simulink model "Quadcopter_NMPC_1"  (R2023a)
settings: Solver=VariableStepAuto  StartTime=0.0  StopTime=10.0  RelTol=1e-3
values from neighbouring files (symbols this model uses):
  Ts = 0.1    [ControlOfQuadrotorUsingNLMPCExample222.m]
undefined symbols (not defined in the file or in its folder): sigbuilder_block, v0, v_set
libraries: mpclib x3, sharedTrackingLibrary x2
settings Model: Creator=Hameed  LastModifiedBy=Hameed
settings DebuggingCC: UnconnectedInputMsg=warning  UnconnectedOutputMsg=warning  UnconnectedLineMsg=warning
settings ModelReferenceCC: EnableRefExpFcnMdlSchedulingChecks=on
settings RTWCC: DLArmComputeVersion=19.05

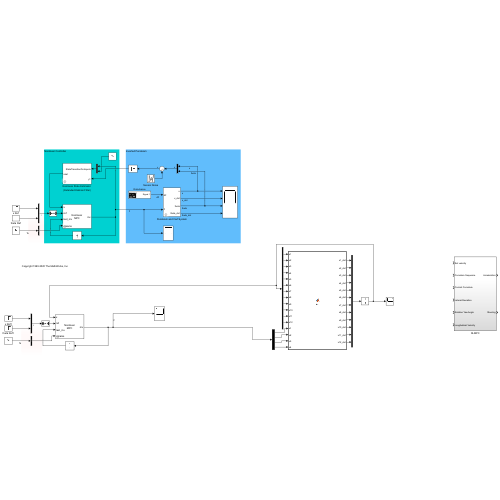
[thumbnail: Simulink's stored preview of the top-level diagram]
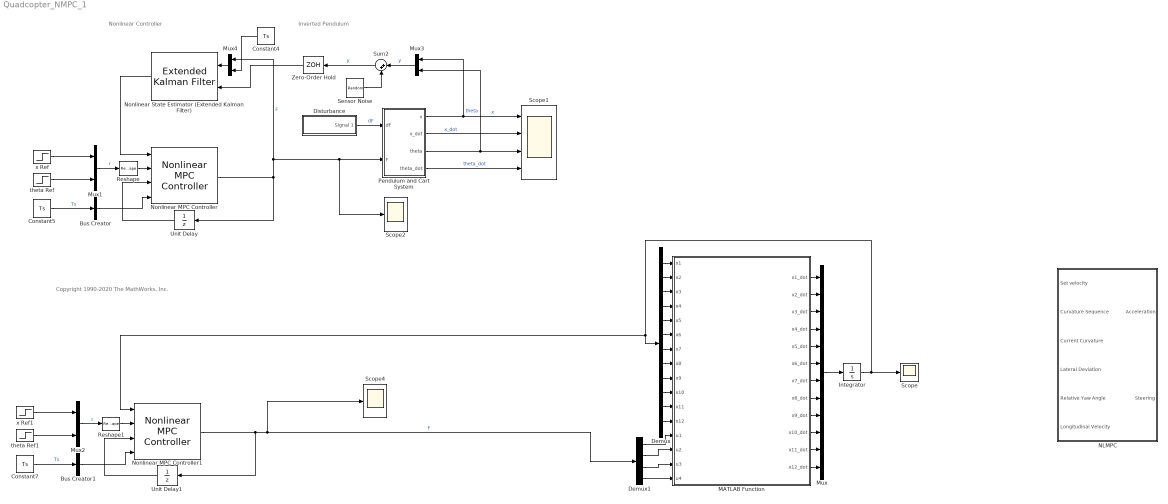
== system Quadcopter_NMPC_1 ==
  note: Inverted Pendulum
  note: Copyright 1990-2020 The MathWorks, Inc.
  note: Nonlinear Controller
  Bus Creator : BusCreator  Inputs=1  OutDataTypeStr=Bus: myBusObject  NonVirtualBus=on
      settings: InheritFromInputs=off
  Bus Creator1 : BusCreator  Inputs=1  OutDataTypeStr=Bus: myBusObject  NonVirtualBus=on
      settings: InheritFromInputs=off
  Constant4 : Constant  Value=Ts
  Constant5 : Constant  Value=Ts
  Constant7 : Constant  Value=Ts
  Demux : Demux  Outputs=12
  Demux1 : Demux
  Disturbance : Subsystem  Tag=STV Subsys  LoadFcn=sigbuilder_block('load');  StartFcn=sigbuilder_block('start');  StopFcn=sigbuilder_block('stop');  ClipboardFcn=sigbuilder_block('clipboard');  mask(Sigbuilder block){tuvar=[0:10]}
      mask help: Simulink:masks:SigbuilderBlock_MD
      mask init:
      | if ~strcmp(get_param(bdroot(gcbh),'SimulationStatus'),'stopped') tuvar = sigbuilder_block('maskInit'); end
      settings: CopyFcn=sigbuilder_block('copy');  DeleteFcn=sigbuilder_block('delete');  ModelCloseFcn=sigbuilder_block('modelClose');  PreSaveFcn=sigbuilder_block('preSave');  PauseFcn=sigbuilder_block('pause');  ContinueFcn=sigbuilder_block('continue');  NameChangeFcn=sigbuilder_block('namechange');  OpenFcn=sigbuilder_block('open',[237 156.75 551.25 355.5 ]);  CloseFcn=sigbuilder_block('close');
      mask Display: plot(0, 0, 100, 100,[2, 2, 32, 32, 2], [68, 8, 8, 68, 68],[32, 2], [38, 38], [32, 19, 2],[53, 60, 44], [32, 17, 17, 2],[16, 16, 31, 31]);txt = getActiveGroup(gcbh);text(2, 100, txt,'verticalAlignment', 'top');
  Integrator : Integrator  InitialCondition=[0;0;0;0;0;0;0;0;0;0;0;0]
  MATLAB Function : MATLAB Function  TreatAsAtomicUnit=on
  Mux : Mux  Inputs=12
  Mux{1..4} (4 alike) : Mux  Inputs=2
  NLMPC : Subsystem  VariantControl=controller_type ==1
  Nonlinear MPC Controller : mpclib/Nonlinear MPC Controller  SCDEnableBlockLinearizationSpecification=on  nlmpcobj=nlobj  UseObjectTs=on  UseMEX=off  md_enabled=off  mvtarget_enabled=off  param_enabled=on  cost_enabled=off  mvseq_enabled=off  stateseq_enabled=off  ovseq_enabled=off  slack_enabled=off  status_enabled=off  ov_min=off  ov_max=off  mv_min=off  mv_max=off  mvrate_min=off  mvrate_max=off  state_min=off  state_max=off  ov_weight=off  mv_weight=off  mvrate_weight=off  ecr_weight=off  nlp_initialize=off
  Nonlinear MPC Controller1 : mpclib/Nonlinear MPC Controller  SCDEnableBlockLinearizationSpecification=on  nlmpcobj=nlobj  UseObjectTs=on  UseMEX=off  md_enabled=off  mvtarget_enabled=off  param_enabled=on  cost_enabled=off  mvseq_enabled=off  stateseq_enabled=off  ovseq_enabled=off  slack_enabled=off  status_enabled=off  ov_min=off  ov_max=off  mv_min=off  mv_max=off  mvrate_min=off  mvrate_max=off  state_min=off  state_max=off  ov_weight=off  mv_weight=off  mvrate_weight=off  ecr_weight=off  nlp_initialize=off
  Nonlinear State Estimator (Extended Kalman Filter) : sharedTrackingLibrary/Extended Kalman Filter  StateTransitionFcn=pendulumStateFcn  HasStateTransitionJacobianFcn=off  HasAdditiveProcessNoise=Additive  ProcessNoise=1e-4*eye(4)  HasTimeVaryingProcessNoise=off  HasStateTransitionFcnExtraArgument=1  InitialState=[0;0;-pi;0]  InitialStateCovariance=1e-4*eye(4)  MeasurementFcn1=pendulumMeasurementFcn  HasMeasurementJacobianFcn1=off  HasMeasurementEnablePort1=off  HasAdditiveMeasurementNoise1=Additive  MeasurementNoise1=1e-4*eye(2)  HasTimeVaryingMeasurementNoise1=off  HasMeasurementFcnExtraArgument1=0  HasMeasurementWrapping1=off  MeasurementFcn2=myMeasurementFcn  HasMeasurementJacobianFcn2=off  HasMeasurementEnablePort2=off  HasAdditiveMeasurementNoise2=Additive  MeasurementNoise2=1  HasTimeVaryingMeasurementNoise2=off  HasMeasurementFcnExtraArgument2=0  HasMeasurementWrapping2=off  MeasurementFcn3=myMeasurementFcn  HasMeasurementJacobianFcn3=off  HasMeasurementEnablePort3=off  HasAdditiveMeasurementNoise3=Additive  MeasurementNoise3=1  HasTimeVaryingMeasurementNoise3=off  HasMeasurementFcnExtraArgument3=0  HasMeasurementWrapping3=off  MeasurementFcn4=myMeasurementFcn  HasMeasurementJacobianFcn4=off  HasMeasurementEnablePort4=off  HasAdditiveMeasurementNoise4=Additive  MeasurementNoise4=1  HasTimeVaryingMeasurementNoise4=off  HasMeasurementFcnExtraArgument4=0  HasMeasurementWrapping4=off  MeasurementFcn5=myMeasurementFcn  HasMeasurementJacobianFcn5=off  HasMeasurementEnablePort5=off  HasAdditiveMeasurementNoise5=Additive  MeasurementNoise5=1  HasTimeVaryingMeasurementNoise5=off  HasMeasurementFcnExtraArgument5=0  HasMeasurementWrapping5=off  EnableMultirate=off  StateTransitionFcnSampleTime=1  MeasurementFcn1SampleTime=1  MeasurementFcn2SampleTime=1  MeasurementFcn3SampleTime=1  MeasurementFcn4SampleTime=1  MeasurementFcn5SampleTime=1  UseCurrentEstimator=on  OutputStateCovariance=off  DataType=double  SampleTime=Ts  NumberOfMeasurements=1
  Pendulum and Cart System : Subsystem  mask{mCartPara=1, mPendPara=1, gPara=9.81, LPara=0.5, KdPara=10, x0=0, theta0=-pi}
      mask prompts: mCartPara "Mass of Cart"; mPendPara "Mass of Pendulum"; gPara "Gravity"; LPara "Length of Pendulum"; KdPara "Friction coefficient of Cart"; x0 "Initial Cart Position"; theta0 "Initial Pendulum Angle"
      mask help: Pendulum and Cart System
      mask init:
      | mCart = str2double(get_param(gcb,'mCartPara'));
      | mPend = str2double(get_param(gcb,'mPendPara'));
      | g = str2double(get_param(gcb,'gPara'));
      | L = str2double(get_param(gcb,'LPara'));
      | Kd = str2double(get_param(gcb,'KdPara'));
  Reshape : Reshape  OutputDimensionality=Row vector (2-D)
  Reshape1 : Reshape  OutputDimensionality=Row vector (2-D)
  Scope : Scope
  Scope1 : Scope  NumInputPorts=4
  Scope2 : Scope
  Scope4 : Scope
  Sensor Noise : UniformRandomNumber  Minimum=-0.01  Maximum=0.01  SampleTime=Ts
  Sum2 : Sum  Inputs=|++
  Unit Delay : UnitDelay  SampleTime=-1  HasFrameUpgradeWarning=on
  Unit Delay1 : UnitDelay  SampleTime=-1  HasFrameUpgradeWarning=on
  Zero-Order Hold : ZeroOrderHold  SampleTime=Ts
  theta Ref : Step  Before=-pi  After=0  SampleTime=0
  theta Ref1 : Step  Before=-pi  After=0  SampleTime=0
  x Ref : Step  Time=10  After=5  SampleTime=0
  x Ref1 : Step  Time=10  After=5  SampleTime=0
  wires:
  Demux1/2 -> MATLAB Function/14(u2)
  Demux1/1 -> MATLAB Function/13(u1)
  Demux1/3 -> MATLAB Function/15(u3)
  Demux1/4 -> MATLAB Function/16(u4)
  Unit Delay1/1 -> Nonlinear MPC Controller1/3
  Mux2/1 -> Reshape1/1  "r"
  Reshape1/1 -> Nonlinear MPC Controller1/2
  Bus Creator1/1 -> Nonlinear MPC Controller1/4
  Constant7/1 -> Bus Creator1/1  "Ts"
  Bus Creator/1 -> Nonlinear MPC Controller/4
  theta Ref/1 -> Mux1/2
  theta Ref1/1 -> Mux2/2
  Pendulum and Cart System/2(x_dot) -> Scope1/2  "x_dot"
  Unit Delay/1 -> Nonlinear MPC Controller/3
  Mux3/1 -> Sum2/1  "y"
  Pendulum and Cart System/1(x) -> Mux3/1, Scope1/1  "x"
  Sensor Noise/1 -> Sum2/2
  Nonlinear MPC Controller/1 -> Unit Delay/1, Pendulum and Cart System/2(F), Scope2/1, Mux4/1  "F"
  Pendulum and Cart System/3(theta) -> Mux3/2, Scope1/3  "theta"
  Sum2/1 -> Zero-Order Hold/1  "y"
  Constant4/1 -> Mux4/2
  Zero-Order Hold/1 -> Nonlinear State Estimator (Extended Kalman Filter)/2
  Demux/7 -> MATLAB Function/7(x7)
  Demux/2 -> MATLAB Function/2(x2)
  Pendulum and Cart System/4(theta_dot) -> Scope1/4  "theta_dot"
  MATLAB Function/3(x3_dot) -> Mux/3
  Disturbance/1(Signal 1) -> Pendulum and Cart System/1(dF)  "dF"
  Demux/12 -> MATLAB Function/12(x12)
  Demux/10 -> MATLAB Function/10(x10)
  MATLAB Function/10(x10_dot) -> Mux/10
  Demux/3 -> MATLAB Function/3(x3)
  MATLAB Function/12(x12_dot) -> Mux/12
  Nonlinear State Estimator (Extended Kalman Filter)/1 -> Nonlinear MPC Controller/1
  Integrator/1 -> Nonlinear MPC Controller1/1, Demux/1, Scope/1
  Demux/1 -> MATLAB Function/1(x1)
  Mux/1 -> Integrator/1
  Mux4/1 -> Nonlinear State Estimator (Extended Kalman Filter)/1
  Constant5/1 -> Bus Creator/1  "Ts"
  MATLAB Function/6(x6_dot) -> Mux/6
  Demux/8 -> MATLAB Function/8(x8)
  Demux/6 -> MATLAB Function/6(x6)
  Demux/11 -> MATLAB Function/11(x11)
  Demux/9 -> MATLAB Function/9(x9)
  Mux1/1 -> Reshape/1  "r"
  Demux/5 -> MATLAB Function/5(x5)
  MATLAB Function/1(x1_dot) -> Mux/1
  Demux/4 -> MATLAB Function/4(x4)
  Nonlinear MPC Controller1/1 -> Unit Delay1/1, Scope4/1, Demux1/1  "F"
  x Ref1/1 -> Mux2/1
  MATLAB Function/4(x4_dot) -> Mux/4
  Reshape/1 -> Nonlinear MPC Controller/2
  MATLAB Function/5(x5_dot) -> Mux/5
  MATLAB Function/9(x9_dot) -> Mux/9
  MATLAB Function/2(x2_dot) -> Mux/2
  MATLAB Function/7(x7_dot) -> Mux/7
  MATLAB Function/8(x8_dot) -> Mux/8
  x Ref/1 -> Mux1/1
  MATLAB Function/11(x11_dot) -> Mux/11

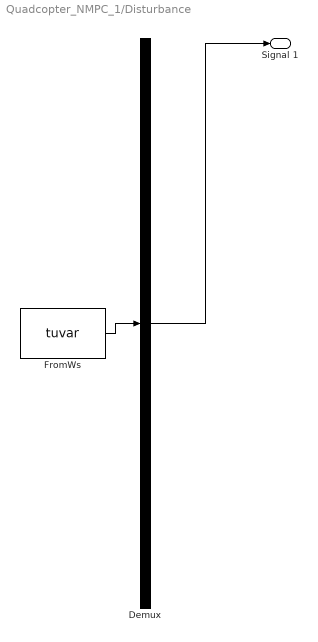
== system Quadcopter_NMPC_1/Disturbance ==
  Demux : Demux  Tag=STV Demux  Outputs=1
      settings: DisplayOption=none
  FromWs : FromWorkspace  Tag=STV FromWs  VariableName=tuvar
      SigBuilderData=|
      | common.afterFinalStr = 'Extrapolate'
      | common.sampleTime = 0
      | dataSet.timeRange = [0 30]
      | dataSet.name = 'Group 1'
      | sbobj.Groups.Name = 'Group 1'
      | sbobj.Groups.Signals.Name = 'Signal 1'
      | sbobj.Groups.Signals.XData = [0 20 20.5 21 30]
      | sbobj.Groups.Signals.YData = [0 0 2 0 0]
      | sbobj.Groups.TimeRange = [0 30]
  Signal 1 : Outport  Tag=STV Outport  VectorParamsAs1DForOutWhenUnconnected=off
  wires:
  FromWs/1 -> Demux/1
  Demux/1 -> Signal 1/1

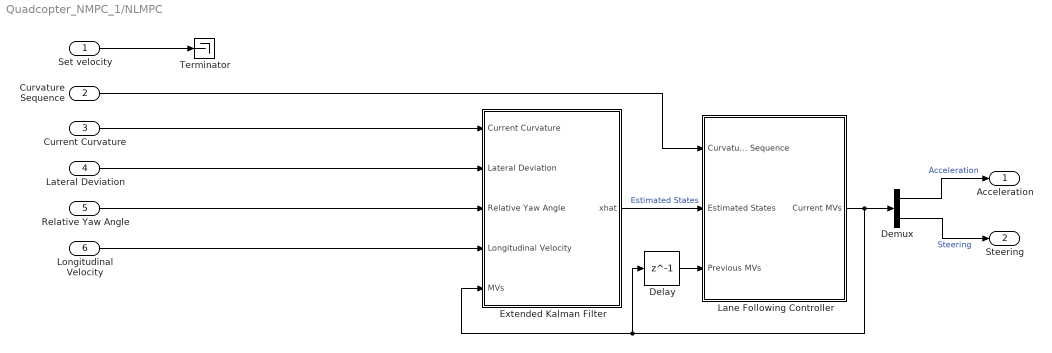
== system Quadcopter_NMPC_1/NLMPC ==
  Set velocity : Inport
  Curvature Sequence : Inport  Port=2
  Current Curvature : Inport  Port=3
  Lateral Deviation : Inport  Port=4
  Relative Yaw Angle : Inport  Port=5
  Longitudinal Velocity : Inport  Port=6
  Delay : Delay  DelayLength=1  InitialCondition=[0.2 0.3]
  Demux : Demux  Outputs=2
  Extended Kalman Filter : Subsystem
  Lane Following Controller : Subsystem
  Terminator : Terminator
  Acceleration : Outport  VectorParamsAs1DForOutWhenUnconnected=off
  Steering : Outport  Port=2  VectorParamsAs1DForOutWhenUnconnected=off
  wires:
  Extended Kalman Filter/1(xhat) -> Lane Following Controller/2(Estimated States)  "Estimated States"
  Lane Following Controller/1(Current MVs) -> Demux/1, Extended Kalman Filter/5(MVs), Delay/1
  Lateral Deviation/1 -> Extended Kalman Filter/2(Lateral Deviation)
  Curvature Sequence/1 -> Lane Following Controller/1(Curvature Sequence)
  Longitudinal Velocity/1 -> Extended Kalman Filter/4(Longitudinal Velocity)
  Delay/1 -> Lane Following Controller/3(Previous MVs)
  Relative Yaw Angle/1 -> Extended Kalman Filter/3(Relative Yaw Angle)
  Current Curvature/1 -> Extended Kalman Filter/1(Current Curvature)
  Set velocity/1 -> Terminator/1
  Demux/2 -> Steering/1  "Steering"
  Demux/1 -> Acceleration/1  "Acceleration"

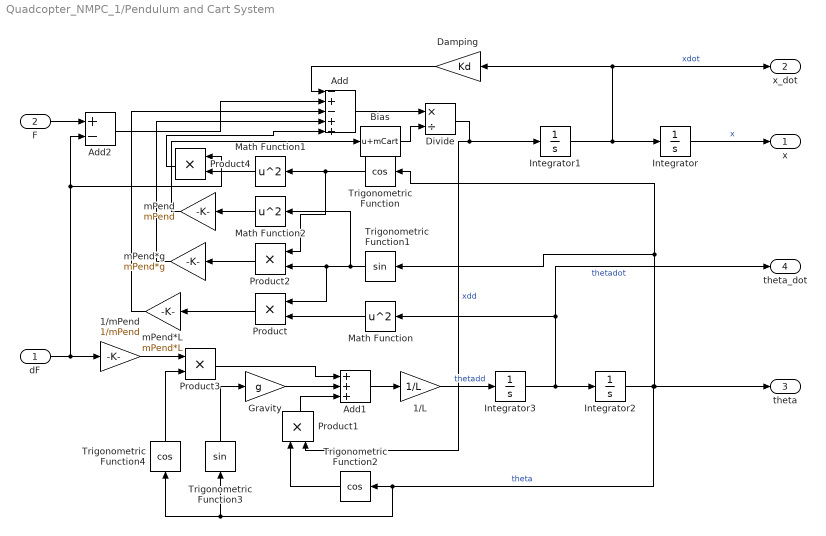
== system Quadcopter_NMPC_1/Pendulum and Cart System ==
  dF : Inport
  F : Inport  Port=2
  1/L : Gain  Gain=1/L
  1/mPend : Gain  Gain=1/mPend
  Add : Sum  Inputs=-+-++
  Add1 : Sum  Inputs=+++
  Add2 : Sum  Inputs=+-
  Bias : Bias  Bias=mCart  SaturateOnIntegerOverflow=off
  Damping : Gain  Gain=Kd
  Divide : Product  Inputs=*/
  Gravity : Gain  Gain=g
  Integrator : Integrator  InitialCondition=x0  ContinuousStateAttributes='x'
  Integrator1 : Integrator  ContinuousStateAttributes='xdot'
  Integrator2 : Integrator  InitialCondition=theta0  ContinuousStateAttributes='theta'
  Integrator3 : Integrator  ContinuousStateAttributes='thetadot'
  Math Function : Math  Operator=square  SignedPower=on
  Math Function1 : Math  Operator=square  SignedPower=on
  Math Function2 : Math  Operator=square  SignedPower=on
  Product{,1..4} (5 alike) : Product
  Trigonometric Function : Trigonometry  Operator=cos
  Trigonometric Function1 : Trigonometry
  Trigonometric Function2 : Trigonometry  Operator=cos
  Trigonometric Function3 : Trigonometry
  Trigonometric Function4 : Trigonometry  Operator=cos
  mPend : Gain  Gain=mPend
  mPend*L : Gain  Gain=mPend*L
  mPend*g : Gain  Gain=mPend*g
  x : Outport  VectorParamsAs1DForOutWhenUnconnected=off
  x_dot : Outport  Port=2  VectorParamsAs1DForOutWhenUnconnected=off
  theta : Outport  Port=3  VectorParamsAs1DForOutWhenUnconnected=off
  theta_dot : Outport  Port=4  VectorParamsAs1DForOutWhenUnconnected=off
  wires:
  mPend/1 -> Bias/1
  Bias/1 -> Divide/2
  Math Function2/1 -> mPend/1
  Product4/1 -> Add/5
  Math Function1/1 -> Product4/2
  mPend*g/1 -> Add/4
  Product1/1 -> Add1/3
  Math Function/1 -> Product/2
  1/L/1 -> Integrator3/1  "thetadd"
  dF/1 -> 1/mPend/1, Product4/1, Add2/2
  1/mPend/1 -> Product3/1
  Trigonometric Function4/1 -> Product3/2
  Damping/1 -> Add/1
  F/1 -> Add2/1
  Trigonometric Function3/1 -> Gravity/1
  Gravity/1 -> Add1/2
  Trigonometric Function/1 -> Math Function1/1, Product2/1
  Integrator3/1 -> Integrator2/1, Math Function/1, theta_dot/1  "thetadot"
  Integrator2/1 -> Trigonometric Function2/1, Trigonometric Function3/1, Trigonometric Function4/1, Trigonometric Function1/1, Trigonometric Function/1, theta/1  "theta"
  Product3/1 -> Add1/1
  Add/1 -> Divide/1
  Divide/1 -> Integrator1/1, Product1/2  "xdd"
  Trigonometric Function2/1 -> Product1/1
  Trigonometric Function1/1 -> Math Function2/1, Product/1, Product2/2
  Integrator/1 -> x/1  "x"
  Integrator1/1 -> Damping/1, x_dot/1, Integrator/1  "xdot"
  Product2/1 -> mPend*g/1
  Add1/1 -> 1/L/1
  Add2/1 -> Add/2
  mPend*L/1 -> Add/3
  Product/1 -> mPend*L/1

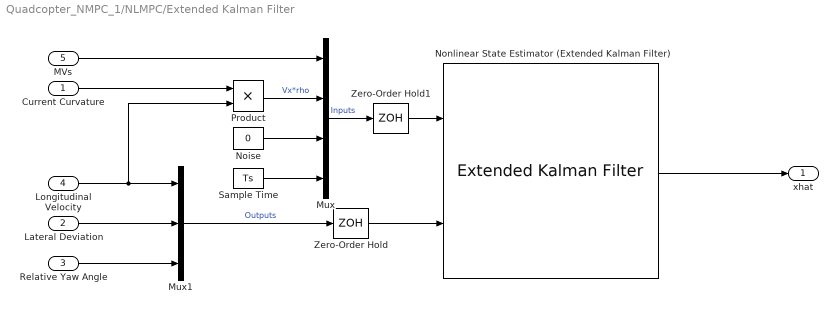
== system Quadcopter_NMPC_1/NLMPC/Extended Kalman Filter ==
  Current Curvature : Inport
  Lateral Deviation : Inport  Port=2
  Relative Yaw Angle : Inport  Port=3
  Longitudinal Velocity : Inport  Port=4
  MVs : Inport  Port=5
  Mux : Mux
  Mux1 : Mux  Inputs=3
  Noise : Constant  Value=0
  Nonlinear State Estimator (Extended Kalman Filter) : sharedTrackingLibrary/Extended Kalman Filter  StateTransitionFcn=LaneFollowingEKFStateFcn11  HasStateTransitionJacobianFcn=off  HasAdditiveProcessNoise=Additive  ProcessNoise=1e-4*eye(7)  HasTimeVaryingProcessNoise=off  HasStateTransitionFcnExtraArgument=1  InitialState=[0 0 v0 0 0 0 0]'  InitialStateCovariance=1e-4*eye(7)  MeasurementFcn1=LaneFollowingEKFMeasFcn11  HasMeasurementJacobianFcn1=off  HasMeasurementEnablePort1=off  HasAdditiveMeasurementNoise1=Additive  MeasurementNoise1=1e-4*eye(3)  HasTimeVaryingMeasurementNoise1=off  HasMeasurementFcnExtraArgument1=0  HasMeasurementWrapping1=off  MeasurementFcn2=myMeasurementFcn  HasMeasurementJacobianFcn2=off  HasMeasurementEnablePort2=off  HasAdditiveMeasurementNoise2=Additive  MeasurementNoise2=1  HasTimeVaryingMeasurementNoise2=off  HasMeasurementFcnExtraArgument2=0  HasMeasurementWrapping2=off  MeasurementFcn3=myMeasurementFcn  HasMeasurementJacobianFcn3=off  HasMeasurementEnablePort3=off  HasAdditiveMeasurementNoise3=Additive  MeasurementNoise3=1  HasTimeVaryingMeasurementNoise3=off  HasMeasurementFcnExtraArgument3=0  HasMeasurementWrapping3=off  MeasurementFcn4=myMeasurementFcn  HasMeasurementJacobianFcn4=off  HasMeasurementEnablePort4=off  HasAdditiveMeasurementNoise4=Additive  MeasurementNoise4=1  HasTimeVaryingMeasurementNoise4=off  HasMeasurementFcnExtraArgument4=0  HasMeasurementWrapping4=off  MeasurementFcn5=myMeasurementFcn  HasMeasurementJacobianFcn5=off  HasMeasurementEnablePort5=off  HasAdditiveMeasurementNoise5=Additive  MeasurementNoise5=1  HasTimeVaryingMeasurementNoise5=off  HasMeasurementFcnExtraArgument5=0  HasMeasurementWrapping5=off  EnableMultirate=off  StateTransitionFcnSampleTime=1  MeasurementFcn1SampleTime=1  MeasurementFcn2SampleTime=1  MeasurementFcn3SampleTime=1  MeasurementFcn4SampleTime=1  MeasurementFcn5SampleTime=1  UseCurrentEstimator=on  OutputStateCovariance=off  DataType=double  SampleTime=Ts  NumberOfMeasurements=1
  Product : Product
  Sample Time : Constant  Value=Ts
  Zero-Order Hold : ZeroOrderHold  SampleTime=Ts
  Zero-Order Hold1 : ZeroOrderHold  SampleTime=Ts
  xhat : Outport  VectorParamsAs1DForOutWhenUnconnected=off
  wires:
  Noise/1 -> Mux/3
  Zero-Order Hold/1 -> Nonlinear State Estimator (Extended Kalman Filter)/2
  MVs/1 -> Mux/1
  Sample Time/1 -> Mux/4
  Nonlinear State Estimator (Extended Kalman Filter)/1 -> xhat/1
  Mux1/1 -> Zero-Order Hold/1  "Outputs"
  Lateral Deviation/1 -> Mux1/2
  Longitudinal Velocity/1 -> Mux1/1, Product/2
  Relative Yaw Angle/1 -> Mux1/3
  Current Curvature/1 -> Product/1
  Product/1 -> Mux/2  "Vx*rho"
  Mux/1 -> Zero-Order Hold1/1  "Inputs"
  Zero-Order Hold1/1 -> Nonlinear State Estimator (Extended Kalman Filter)/1

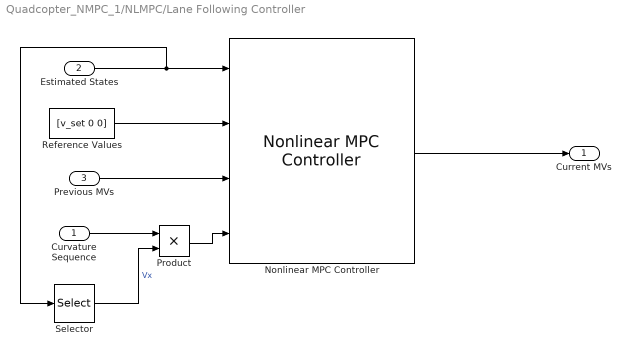
== system Quadcopter_NMPC_1/NLMPC/Lane Following Controller ==
  Curvature Sequence : Inport
  Estimated States : Inport  Port=2
  Previous MVs : Inport  Port=3
  Nonlinear MPC Controller : mpclib/Nonlinear MPC Controller  SCDEnableBlockLinearizationSpecification=on  nlmpcobj=nlobj  UseObjectTs=on  TsControl=Ts  UseMEX=off  md_enabled=on  mvtarget_enabled=off  param_enabled=off  cost_enabled=off  mvseq_enabled=off  stateseq_enabled=off  ovseq_enabled=off  slack_enabled=off  status_enabled=off  ov_min=off  ov_max=off  mv_min=off  mv_max=off  mvrate_min=off  mvrate_max=off  state_min=off  state_max=off  ov_weight=off  mv_weight=off  mvrate_weight=off  ecr_weight=off  nlp_initialize=off
  Product : Product
  Reference Values : Constant  Value=[v_set 0 0]  VectorParams1D=off
  Selector : Selector  InputPortWidth=7  IndexOptions=Index vector (dialog)  Indices=[3]  OutputSizes=1
  Current MVs : Outport  VectorParamsAs1DForOutWhenUnconnected=off
  wires:
  Previous MVs/1 -> Nonlinear MPC Controller/3
  Reference Values/1 -> Nonlinear MPC Controller/2
  Estimated States/1 -> Selector/1, Nonlinear MPC Controller/1
  Nonlinear MPC Controller/1 -> Current MVs/1
  Selector/1 -> Product/2  "Vx"
  Curvature Sequence/1 -> Product/1
  Product/1 -> Nonlinear MPC Controller/4

== matlab function Quadcopter_NMPC_1/MATLAB Function ==
  data: x1 input; x1_dot output; x2 input; x3 input; x4 input; x5 input; x6 input; x7 input; x8 input; x9 input; x10 input; x11 input; x12 input; u1 input; u2 input; u3 input; u4 input; x2_dot output; x3_dot output; x4_dot output; x5_dot output; x6_dot output; x7_dot output; x8_dot output; x9_dot output; x10_dot output; x11_dot output; x12_dot output
function [x1_dot,x2_dot,x3_dot,x4_dot,x5_dot,x6_dot,x7_dot,x8_dot,x9_dot,x10_dot,x11_dot,x12_dot]= fcn(x1,x2,x3,x4,x5,x6,x7,x8,x9,x10,x11,x12,u1,u2,u3,u4)
% x=x1;
% y=x2,
% z=x3
% phi=x4;
% theta=x5;
% sai=x6;
% x_dot=x7;
% y_dot=x8,
% z_dot=x9
% phi_dot=x10;
% theta_dot=x11;
% sai_dot=x12;

Ixx= 1.2; 
Iyy= 1.2;
Izz= 2.3;
k= 1;
l= 0.25;
m= 2;
b= 0.2;
g= 9.81;

T = k*(u1+u2+u3+u4);
x789= -g*[0;0;1]+(T/m)*[sin(x6)*sin(x5)*sin(x4)+sin(x6)*sin(x4);cos(x6)*cos(x5)*cos(x4)-cos(x6)*cos(x4);cos(x5)*cos(x4)];

tB= [l*k*(-u2 + u4);l*k*(-u1 + u3);b*(-u1+u2-u3+u4)];


C11=0
C12=(Iyy-Izz)*(x7*cos(x4)*sin(x4)+x12*sin(x4)^2*cos(x5))+(Izz-Iyy)*x12*cos(x4)^2*cos(x5)-Ixx*x12*cos(x5);
C13=(Izz-Iyy)*(x12*cos(x4)*sin(x4)*cos(x5)^2);
C21=(Izz-Iyy)*(x7*cos(x4)*sin(x4)+x12*sin(x4)*cos(x5))+(Iyy-Izz)*x12*cos(x4)^2*cos(x5)-Ixx*x12*cos(x5);
C22=(Izz-Iyy)*x10*cos(x4)*sin(x4);
C23= -Ixx*x12*sin(x5)*cos(x5)+Iyy*x12*sin(x4)^2*sin(x5)*cos(x5)+ Izz*x12*cos(x4)^2*sin(x5)*cos(x5);
C31=(Iyy-Izz)*(x12*cos(x5)^2*sin(x4)*cos(x4))-Ixx*x11*cos(x5);
C32= (Izz-Iyy)*(x11*cos(x4)*sin(x4)*sin(x5)+x10*sin(x4)^2*cos(x5))+(Iyy-Izz)*x10*cos(x4)^2*cos(x5)+Ixx*x12*cos(x5)*cos(x5)-Iyy*x12*sin(x10)^2*sin(x5)*cos(x5)-Izz*x12*cos(x10)^2*sin(x5)*cos(x5);
C33=(Iyy-Izz)*x10*cos(x4)*sin(x4)*cos(x5)^2-Iyy*x11*sin(x4)^2*cos(x5)*sin(x5)-Izz*x11*cos(x4)^2*cos(x5)*sin(x5)+Ixx*x11*cos(x5)*sin(x5);
Cnndot=[C11 C12 C13;C21 C22 C23;C31 C32 C33];

%ndot=[x10_dot;x11_dot;x12_dot];
ndot=[x10;x11;x12];


W = [1, 0, -sin(x5);
    0, cos(x4), cos(x5)*sin(x4);
    0, -sin(x4), cos(x5)*cos(x4)];
I = [Ixx,0,0;0,Iyy,0;0,0,Izz];
J = W.'*I*W;

x101112= inv(J)*(tB-Cnndot*ndot);

x1_dot=x7;
x2_dot=x8;
x3_dot=x9;
x4_dot=x10;
x5_dot=x11;
x6_dot=x12;
x7_dot=x789(1);
x8_dot=x789(2);
x9_dot=x789(3);
x10_dot=x101112(1);
x11_dot=x101112(2);
x12_dot=x101112(3);


%y=u;
